simulink model "torqueBalancingStandup"  (Simulink 9.1)
settings: Solver=FixedStepDiscrete  StartTime=0.0  StopTime="Config.SIMULATION_TIME "  FixedStep=Config.Ts  RelTol=1e-3  EnableMultiTasking=on
InitFcn:
  | cd(fileparts(which(bdroot)));
  | initTorqueBalancingPHRIStandup;
StopFcn:
  | cd(fileparts(which(bdroot)));
  | stopTorqueBalancingPHRIStandup;
undefined symbols (not defined in the file or in its folder): bVectorConstraintsFeet, bVectorConstraintsLegs, Config, ConstraintsMatrixFeet, ConstraintsMatrixLegs, Gain, HUMAN_DOF_FOR_SIMULINK, Reg, ROBOT_DOF, ROBOT_DOF_FOR_SIMULINK, Sat, Sm
libraries: WBToolboxLibrary x127, simulink x4
(part 2 of 3)

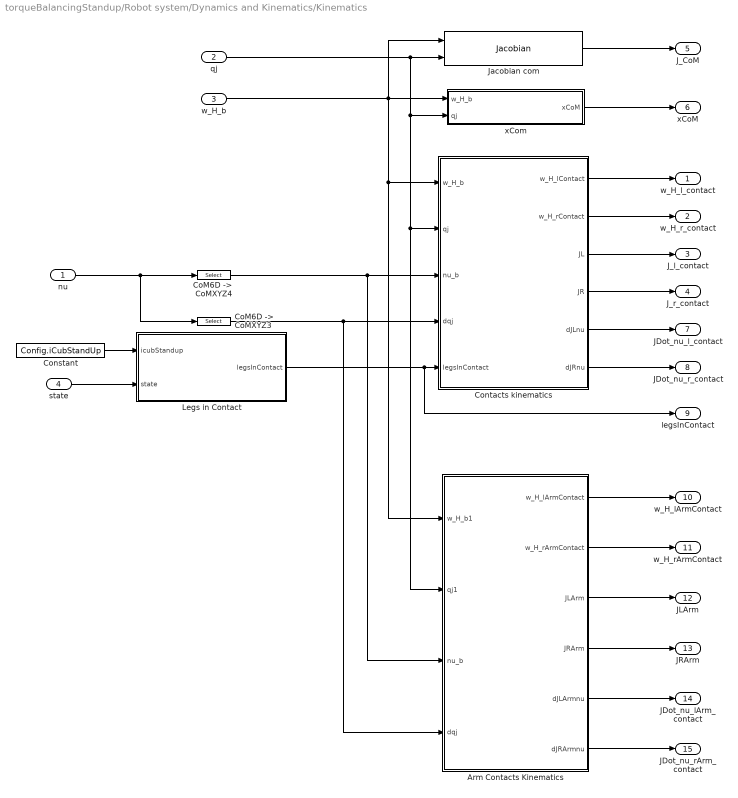
== system torqueBalancingStandup/Robot system/Dynamics and Kinematics/Kinematics ==
  nu : Inport
  qj : Inport  Port=2
  w_H_b : Inport  Port=3
  "state " : Inport  Port=4
  Arm Contacts Kinematics : Subsystem
  "CoM6D ->  CoMXYZ3" : Selector  InputPortWidth=6+ROBOT_DOF  IndexOptions=Index vector (dialog)  Indices=[7:6+ROBOT_DOF]  OutputSizes=1
  "CoM6D ->  CoMXYZ4" : Selector  InputPortWidth=6+ROBOT_DOF  IndexOptions=Index vector (dialog)  Indices=[1 2 3 4 5 6]  OutputSizes=1
  Constant : Constant  Value=Config.iCubStandUp
  Contacts kinematics : Subsystem
  Jacobian com : WBToolboxLibrary/wholeBodyModel/Jacobians/Jacobian  frameName=Frames.COM
      settings: SourceProductName=Whole Body Toolbox
  Legs in Contact : MATLAB Function  TreatAsAtomicUnit=on
  xCom : Subsystem
  w_H_l_contact : Outport
  w_H_r_contact : Outport  Port=2
  J_l_contact : Outport  Port=3
  J_r_contact : Outport  Port=4
  J_CoM : Outport  Port=5
  xCoM : Outport  Port=6
  JDot_nu_l_contact : Outport  Port=7
  JDot_nu_r_contact : Outport  Port=8
  legsInContact : Outport  Port=9
  w_H_lArmContact : Outport  Port=10
  w_H_rArmContact : Outport  Port=11
  JLArm : Outport  Port=12
  JRArm : Outport  Port=13
  JDot_nu_lArm_contact : Outport  Port=14
  JDot_nu_rArm_contact : Outport  Port=15
  wires:
  nu/1 -> "CoM6D ->  CoMXYZ3"/1, "CoM6D ->  CoMXYZ4"/1
  w_H_b/1 -> Arm Contacts Kinematics/1(w_H_b1), Contacts kinematics/1(w_H_b), xCom/1(w_H_b), Jacobian com/1
  qj/1 -> Jacobian com/2, Arm Contacts Kinematics/2(qj1), Contacts kinematics/2(qj), xCom/2(qj)
  Jacobian com/1 -> J_CoM/1
  xCom/1(xCoM) -> xCoM/1
  "state "/1 -> Legs in Contact/2(state)
  Constant/1 -> Legs in Contact/1(icubStandup)
  "CoM6D ->  CoMXYZ3"/1 -> Arm Contacts Kinematics/4(dqj), Contacts kinematics/4(dqj)
  "CoM6D ->  CoMXYZ4"/1 -> Arm Contacts Kinematics/3(nu_b), Contacts kinematics/3(nu_b)
  Legs in Contact/1(legsInContact) -> Contacts kinematics/5(legsInContact), legsInContact/1
  Contacts kinematics/1(w_H_lContact) -> w_H_l_contact/1
  Contacts kinematics/2(w_H_rContact) -> w_H_r_contact/1
  Contacts kinematics/5(dJLnu) -> JDot_nu_l_contact/1
  Contacts kinematics/6(dJRnu) -> JDot_nu_r_contact/1
  Contacts kinematics/3(JL) -> J_l_contact/1
  Contacts kinematics/4(JR) -> J_r_contact/1
  Arm Contacts Kinematics/4(JRArm) -> JRArm/1
  Arm Contacts Kinematics/5(dJLArmnu) -> JDot_nu_lArm_contact/1
  Arm Contacts Kinematics/3(JLArm) -> JLArm/1
  Arm Contacts Kinematics/1(w_H_lArmContact) -> w_H_lArmContact/1
  Arm Contacts Kinematics/6(dJRArmnu) -> JDot_nu_rArm_contact/1
  Arm Contacts Kinematics/2(w_H_rArmContact) -> w_H_rArmContact/1

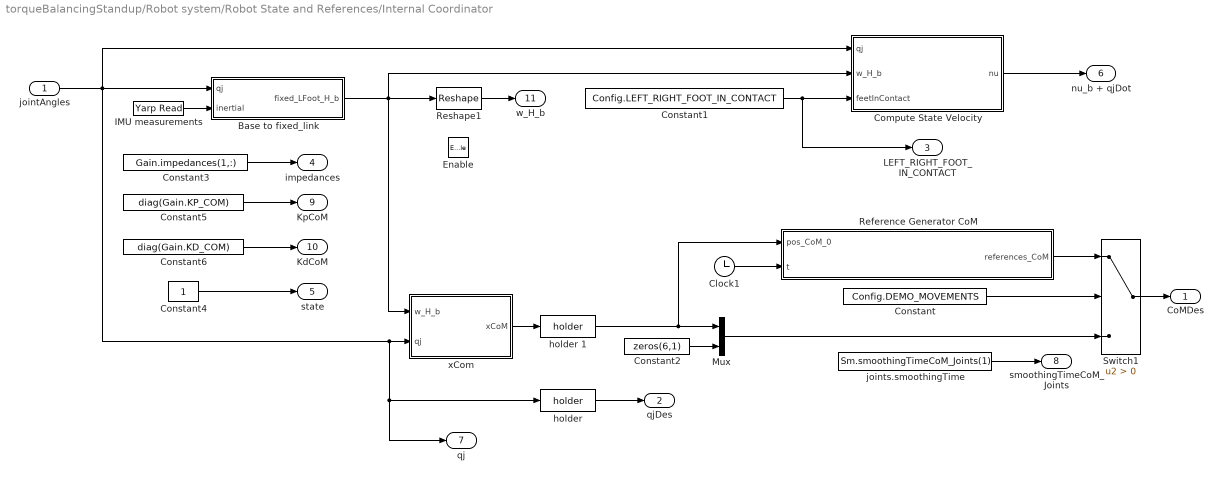
== system torqueBalancingStandup/Robot system/Robot State and References/Internal Coordinator ==
  jointAngles : Inport
  Enable : EnablePort
  Base to fixed_link : Subsystem
  Clock1 : Clock
  Compute State Velocity : Subsystem
  Constant : Constant  Value=Config.DEMO_MOVEMENTS
  Constant1 : Constant  Value=Config.LEFT_RIGHT_FOOT_IN_CONTACT
  Constant2 : Constant  Value=zeros(6,1)
  Constant3 : Constant  Value=Gain.impedances(1,:)
  Constant4 : Constant
  Constant5 : Constant  Value=diag(Gain.KP_COM)
  Constant6 : Constant  Value=diag(Gain.KD_COM)
  IMU measurements : WBToolboxLibrary/Utilities/Yarp Read  portName=Ports.IMU  signalSize=12  timeout=0.5  blocking=off  timestamp=off  autoconnect=on  errorOnConnection=on
      settings: SourceProductName=Whole Body Toolbox
  Mux : Mux  Inputs=2
  Reference Generator CoM : MATLAB Function  TreatAsAtomicUnit=on
  Reshape1 : Reshape  OutputDimensions=[4;4]
  Switch1 : Switch  Criteria=u2 > Threshold
  "holder " : WBToolboxLibrary/Utilities/holder 
      settings: SourceProductName=Whole Body Toolbox
  holder 1 : WBToolboxLibrary/Utilities/holder 
      settings: SourceProductName=Whole Body Toolbox
  joints.smoothingTime : Constant  Value=Sm.smoothingTimeCoM_Joints(1)
  xCom : Subsystem
  CoMDes : Outport
  qjDes : Outport  Port=2
  LEFT_RIGHT_FOOT_IN_CONTACT : Outport  Port=3
  impedances : Outport  Port=4
  state : Outport  Port=5
  nu_b + qjDot : Outport  Port=6
  qj : Outport  Port=7
  smoothingTimeCoM_Joints : Outport  Port=8
  KpCoM : Outport  Port=9
  KdCoM : Outport  Port=10
  w_H_b : Outport  Port=11
  wires:
  Constant/1 -> Switch1/2
  "holder "/1 -> qjDes/1
  Switch1/1 -> CoMDes/1
  Mux/1 -> Switch1/3
  Constant2/1 -> Mux/2
  Constant3/1 -> impedances/1
  Constant4/1 -> state/1
  Compute State Velocity/1(nu) -> nu_b + qjDot/1
  holder 1/1 -> Reference Generator CoM/1(pos_CoM_0), Mux/1
  Base to fixed_link/1(fixed_LFoot_H_b) -> Compute State Velocity/2(w_H_b), xCom/1(w_H_b), Reshape1/1
  xCom/1(xCoM) -> holder 1/1
  joints.smoothingTime/1 -> smoothingTimeCoM_Joints/1
  jointAngles/1 -> Compute State Velocity/1(qj), Base to fixed_link/1(qj), qj/1, "holder "/1, xCom/2(qj)
  Constant5/1 -> KpCoM/1
  Constant6/1 -> KdCoM/1
  Reshape1/1 -> w_H_b/1
  Constant1/1 -> Compute State Velocity/3("feetInContact "), LEFT_RIGHT_FOOT_IN_CONTACT/1
  IMU measurements/1 -> Base to fixed_link/2(inertial)
  Clock1/1 -> Reference Generator CoM/2(t)
  Reference Generator CoM/1(references_CoM) -> Switch1/1

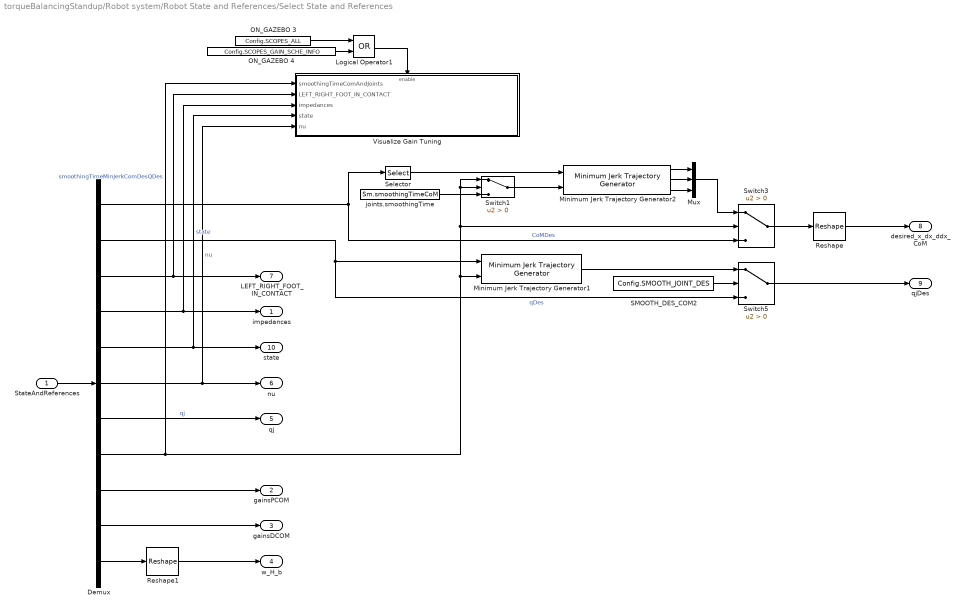
== system torqueBalancingStandup/Robot system/Robot State and References/Select State and References ==
  StateAndReferences : Inport
  Demux : Demux  Outputs=[9,ROBOT_DOF,2,ROBOT_DOF,1,ROBOT_DOF+6,ROBOT_DOF,1,3,3,16]
  Logical Operator1 : Logic  Operator=OR  AllPortsSameDT=off  OutDataTypeStr=boolean
  Minimum Jerk Trajectory Generator1 : WBToolboxLibrary/Utilities/Minimum Jerk Trajectory Generator  externalSettlingTime=on  settlingTime=1  sampleTime=Config.Ts  resetOnSettlingTime=off  firstDerivatives=off  secondDerivatives=off  explicitInitialValue=off
      settings: SourceProductName=Whole Body Toolbox
  Minimum Jerk Trajectory Generator2 : WBToolboxLibrary/Utilities/Minimum Jerk Trajectory Generator  externalSettlingTime=on  settlingTime=0.1  sampleTime=Config.Ts  resetOnSettlingTime=off  firstDerivatives=on  secondDerivatives=on  explicitInitialValue=off
      settings: SourceProductName=Whole Body Toolbox
  Mux : Mux  Inputs=3
  ON_GAZEBO 3 : Constant  Value=Config.SCOPES_ALL
  ON_GAZEBO 4 : Constant  Value=Config.SCOPES_GAIN_SCHE_INFO
  Reshape : Reshape  OutputDimensionality=Customize  OutputDimensions=[3,3]
  Reshape1 : Reshape  OutputDimensionality=Customize  OutputDimensions=[4;4]
  SMOOTH_DES_COM2 : Constant  Value=Config.SMOOTH_JOINT_DES
  Selector : Selector  InputPortWidth=9  IndexOptions=Index vector (dialog)  Indices=[1 2 3]  OutputSizes=1
  Switch1 : Switch  Criteria=u2 > Threshold
  Switch3 : Switch  Criteria=u2 > Threshold
  Switch5 : Switch  Criteria=u2 > Threshold
  "Visualize Gain Tuning  " : Subsystem
  joints.smoothingTime : Constant  Value=Sm.smoothingTimeCoM
  impedances : Outport
  gainsPCOM : Outport  Port=2
  gainsDCOM : Outport  Port=3
  w_H_b : Outport  Port=4
  qj : Outport  Port=5
  nu : Outport  Port=6
  LEFT_RIGHT_FOOT_IN_CONTACT : Outport  Port=7
  desired_x_dx_ddx_CoM : Outport  Port=8
  qjDes : Outport  Port=9
  state : Outport  Port=10
  wires:
  Reshape/1 -> desired_x_dx_ddx_CoM/1
  Minimum Jerk Trajectory Generator2/1 -> Mux/1
  Minimum Jerk Trajectory Generator2/2 -> Mux/2
  Switch3/1 -> Reshape/1
  Minimum Jerk Trajectory Generator2/3 -> Mux/3
  SMOOTH_DES_COM2/1 -> Switch5/2
  Switch5/1 -> qjDes/1
  Demux/7 -> qj/1  "qj"
  Demux/11 -> Reshape1/1
  Demux/5 -> "Visualize Gain Tuning  "/4(state), state/1  "state"
  Demux/8 -> Switch1/1, Switch1/2, Switch3/2, Minimum Jerk Trajectory Generator1/2, "Visualize Gain Tuning  "/1(smoothingTimeComAndJoints)  "smoothingTimeMinJerkComDesQDes"
  Mux/1 -> Switch3/1
  Selector/1 -> Minimum Jerk Trajectory Generator2/1
  Demux/2 -> Switch5/3, Minimum Jerk Trajectory Generator1/1  "qDes"
  Minimum Jerk Trajectory Generator1/1 -> Switch5/1
  Demux/6 -> "Visualize Gain Tuning  "/5(nu), nu/1  "nu"
  StateAndReferences/1 -> Demux/1
  Demux/4 -> "Visualize Gain Tuning  "/3(impedances), impedances/1
  Demux/3 -> "Visualize Gain Tuning  "/2(LEFT_RIGHT_FOOT_IN_CONTACT), LEFT_RIGHT_FOOT_IN_CONTACT/1
  Demux/9 -> gainsPCOM/1
  Demux/10 -> gainsDCOM/1
  Demux/1 -> Selector/1, Switch3/3  "CoMDes"
  Reshape1/1 -> w_H_b/1
  ON_GAZEBO 4/1 -> Logical Operator1/2
  ON_GAZEBO 3/1 -> Logical Operator1/1
  Logical Operator1/1 -> "Visualize Gain Tuning  "/Enable
  Switch1/1 -> Minimum Jerk Trajectory Generator2/2
  joints.smoothingTime/1 -> Switch1/3

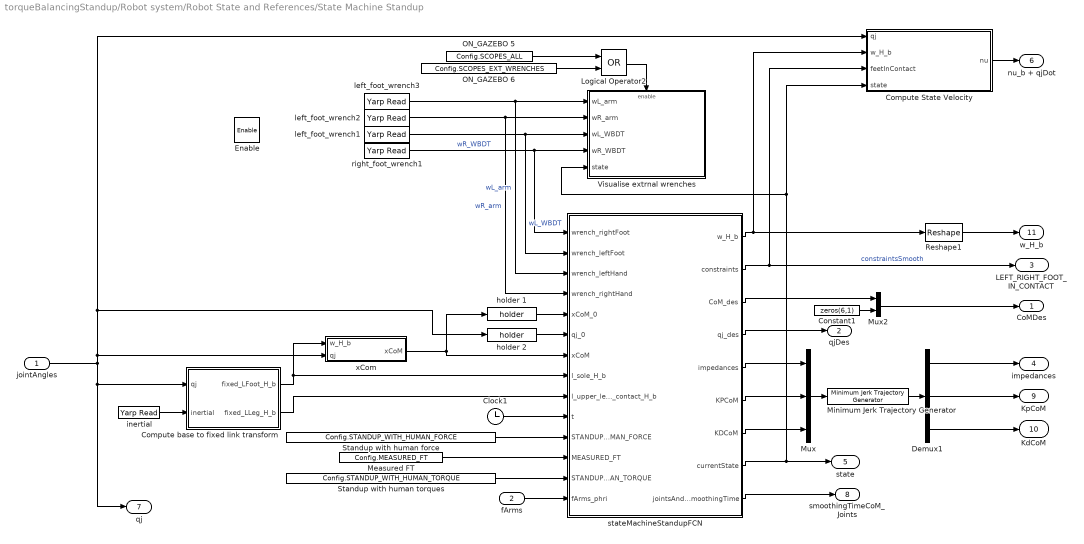
== system torqueBalancingStandup/Robot system/Robot State and References/State Machine Standup ==
  jointAngles : Inport
  fArms : Inport  Port=2
  Enable : EnablePort
  Clock1 : Clock
  Compute State Velocity : Subsystem
  Compute base to fixed link transform : Subsystem
  Constant1 : Constant  Value=zeros(6,1)
  Demux1 : Demux  Outputs=[ROBOT_DOF,3,3]
  Logical Operator2 : Logic  Operator=OR  AllPortsSameDT=off  OutDataTypeStr=boolean
  Measured FT : Constant  Value=Config.MEASURED_FT
  Minimum Jerk Trajectory Generator : WBToolboxLibrary/Utilities/Minimum Jerk Trajectory Generator  externalSettlingTime=off  settlingTime=Gain.SmoothingTimeGainScheduling  sampleTime=Config.Ts  resetOnSettlingTime=off  firstDerivatives=off  secondDerivatives=off  explicitInitialValue=off
      settings: SourceProductName=Whole Body Toolbox
  Mux : Mux  Inputs=3
  Mux2 : Mux  Inputs=2
  ON_GAZEBO 5 : Constant  Value=Config.SCOPES_ALL
  ON_GAZEBO 6 : Constant  Value=Config.SCOPES_EXT_WRENCHES
  Reshape1 : Reshape  OutputDimensions=[4;4]
  Standup with human force : Constant  Value=Config.STANDUP_WITH_HUMAN_FORCE
  Standup with human torques : Constant  Value=Config.STANDUP_WITH_HUMAN_TORQUE
  Visualise extrnal wrenches : Subsystem
  holder 1 : WBToolboxLibrary/Utilities/holder 
      settings: SourceProductName=Whole Body Toolbox
  holder 2 : WBToolboxLibrary/Utilities/holder 
      settings: SourceProductName=Whole Body Toolbox
  inertial : WBToolboxLibrary/Utilities/Yarp Read  portName=Ports.IMU  signalSize=12  timeout=0.5  blocking=off  timestamp=off  autoconnect=on  errorOnConnection=off
      settings: SourceProductName=Whole Body Toolbox
  left_foot_wrench1 : WBToolboxLibrary/Utilities/Yarp Read  portName=Ports.WBD_LEFTLEG_EE  signalSize=6  timeout=0.5  blocking=off  timestamp=off  autoconnect=on  errorOnConnection=on
      settings: SourceProductName=Whole Body Toolbox
  left_foot_wrench2 : WBToolboxLibrary/Utilities/Yarp Read  portName=Ports.RIGHT_ARM  signalSize=6  timeout=0.5  blocking=off  timestamp=off  autoconnect=on  errorOnConnection=on
      settings: SourceProductName=Whole Body Toolbox
  left_foot_wrench3 : WBToolboxLibrary/Utilities/Yarp Read  portName=Ports.LEFT_ARM  signalSize=6  timeout=0.5  blocking=off  timestamp=off  autoconnect=on  errorOnConnection=on
      settings: SourceProductName=Whole Body Toolbox
  right_foot_wrench1 : WBToolboxLibrary/Utilities/Yarp Read  portName=Ports.WBD_RIGHTLEG_EE  signalSize=6  timeout=0.5  blocking=off  timestamp=off  autoconnect=on  errorOnConnection=on
      settings: SourceProductName=Whole Body Toolbox
  stateMachineStandupFCN : MATLAB Function  TreatAsAtomicUnit=on
  xCom : Subsystem
  CoMDes : Outport
  qjDes : Outport  Port=2
  LEFT_RIGHT_FOOT_IN_CONTACT : Outport  Port=3
  impedances : Outport  Port=4
  state : Outport  Port=5
  nu_b + qjDot : Outport  Port=6
  qj : Outport  Port=7
  smoothingTimeCoM_Joints : Outport  Port=8
  KpCoM : Outport  Port=9
  KdCoM : Outport  Port=10
  w_H_b : Outport  Port=11
  wires:
  xCom/1(xCoM) -> holder 1/1, stateMachineStandupFCN/7(xCoM)
  stateMachineStandupFCN/4(qj_des) -> qjDes/1
  stateMachineStandupFCN/3(CoM_des) -> Mux2/1
  Mux2/1 -> CoMDes/1
  Constant1/1 -> Mux2/2
  stateMachineStandupFCN/8(currentState) -> Visualise extrnal wrenches/5(state), Compute State Velocity/4("state "), state/1
  stateMachineStandupFCN/2(constraints) -> LEFT_RIGHT_FOOT_IN_CONTACT/1, Compute State Velocity/3("feetInContact ")  "constraintsSmooth"
  stateMachineStandupFCN/1(w_H_b) -> Reshape1/1, Compute State Velocity/2(w_H_b)
  Compute State Velocity/1(nu) -> nu_b + qjDot/1
  stateMachineStandupFCN/9(jointsAndCoMSmoothingTime) -> smoothingTimeCoM_Joints/1
  stateMachineStandupFCN/6(KPCoM) -> Mux/2
  Demux1/3 -> KdCoM/1
  stateMachineStandupFCN/7(KDCoM) -> Mux/3
  stateMachineStandupFCN/5(impedances) -> Mux/1
  Mux/1 -> Minimum Jerk Trajectory Generator/1
  Minimum Jerk Trajectory Generator/1 -> Demux1/1
  Demux1/1 -> impedances/1
  Demux1/2 -> KpCoM/1
  jointAngles/1 -> Compute State Velocity/1(qj), holder 2/1, xCom/2(qj), qj/1, Compute base to fixed link transform/1(qj)
  Compute base to fixed link transform/1(fixed_LFoot_H_b) -> xCom/1(w_H_b), stateMachineStandupFCN/8(l_sole_H_b)
  Compute base to fixed link transform/2(fixed_LLeg_H_b) -> stateMachineStandupFCN/9(l_upper_leg_contact_H_b)
  inertial/1 -> Compute base to fixed link transform/2(inertial)
  Reshape1/1 -> w_H_b/1
  right_foot_wrench1/1 -> stateMachineStandupFCN/1(wrench_rightFoot), Visualise extrnal wrenches/4(wR_WBDT)  "wR_WBDT"
  left_foot_wrench1/1 -> stateMachineStandupFCN/2(wrench_leftFoot), Visualise extrnal wrenches/3(wL_WBDT)  "wL_WBDT"
  Logical Operator2/1 -> Visualise extrnal wrenches/Enable
  ON_GAZEBO 5/1 -> Logical Operator2/1
  ON_GAZEBO 6/1 -> Logical Operator2/2
  left_foot_wrench2/1 -> stateMachineStandupFCN/4(wrench_rightHand), Visualise extrnal wrenches/2(wR_arm)  "wR_arm"
  left_foot_wrench3/1 -> stateMachineStandupFCN/3(wrench_leftHand), Visualise extrnal wrenches/1(wL_arm)  "wL_arm"
  holder 1/1 -> stateMachineStandupFCN/5(xCoM_0)
  holder 2/1 -> stateMachineStandupFCN/6(qj_0)
  Clock1/1 -> stateMachineStandupFCN/10(t)
  Measured FT/1 -> stateMachineStandupFCN/12(MEASURED_FT)
  fArms/1 -> stateMachineStandupFCN/14(fArms_phri)
  Standup with human force/1 -> stateMachineStandupFCN/11(STANDUP_WITH_HUMAN_FORCE)
  Standup with human torques/1 -> stateMachineStandupFCN/13(STANDUP_WITH_HUMAN_TORQUE)

== system torqueBalancingStandup/Robot system/controller_QP/Compute angular momentum integral ==
  qjDes : Inport
  qj : Inport  Port=2
  constraints : Inport  Port=3
  state : Inport  Port=4
  Centroidal Momentum : WBToolboxLibrary/wholeBodyModel/Dynamics/Centroidal Momentum
      settings: SourceProductName=Whole Body Toolbox
  Compute base to fixed link transform : Subsystem
  Constant : Constant  Value=Config.iCubStandUp
  Fixed Links Jacobians : Subsystem
  Legs in Contact : MATLAB Function  TreatAsAtomicUnit=on
  References for H : MATLAB Function  TreatAsAtomicUnit=on
  Selector : Selector  InputPortWidth=6  IndexOptions=Index vector (dialog)  Indices=[4 5 6]  OutputSizes=1
  Sum : Sum  Inputs=|-+
  Switch : Switch  Criteria=u2 > Threshold  Threshold=0.1
  inertial : WBToolboxLibrary/Utilities/Yarp Read  portName=Ports.IMU  signalSize=12  timeout=0.5  blocking=off  timestamp=off  autoconnect=on  errorOnConnection=on
      settings: SourceProductName=Whole Body Toolbox
  intHw : Outport
  wires:
  qjDes/1 -> Sum/1, Compute base to fixed link transform/1(qj), Fixed Links Jacobians/2(qj), Centroidal Momentum/2
  qj/1 -> Sum/2
  Sum/1 -> Centroidal Momentum/4, References for H/1(qjErr)
  References for H/1(nu_b_equivalent) -> Centroidal Momentum/3
  Fixed Links Jacobians/1(J_LeftFixed) -> References for H/2(JL)
  Centroidal Momentum/1 -> Selector/1
  Selector/1 -> intHw/1
  Fixed Links Jacobians/2(J_RIghtFixed) -> References for H/3(JR)
  constraints/1 -> References for H/4(activeFeetConstraints)
  Switch/1 -> Centroidal Momentum/1, Fixed Links Jacobians/3(w_H_b)
  inertial/1 -> Compute base to fixed link transform/2(inertial)
  state/1 -> Legs in Contact/2(state)
  Constant/1 -> Legs in Contact/1(icubStandup)
  Legs in Contact/1(legsInContact) -> Fixed Links Jacobians/1("legsInContact "), Switch/2
  Compute base to fixed link transform/1(fixed_LLeg_H_b) -> Switch/1
  Compute base to fixed link transform/2(fixed_LFoot_H_b) -> Switch/3

== system torqueBalancingStandup/Robot system/controller_QP/Compute joint torques ==
  LEFT_RIGHT_FOOT_IN_CONTACT : Inport
  tauModel : Inport  Port=2
  Sigma : Inport  Port=3
  NA : Inport  Port=4
  fHDes : Inport  Port=5
  HessianMatrixQP1Foot : Inport  Port=6
  gradientQP1Foot : Inport  Port=7
  ConstraintsMatrixQP1Foot : Inport  Port=8
  bVectorConstraintsQP1Foot : Inport  Port=9
  HessianMatrixQP2Feet : Inport  Port=10
  gradientQP2Feet : Inport  Port=11
  ConstraintsMatrixQP2Feet : Inport  Port=12
  bVectorConstraintsQp2Feet : Inport  Port=13
  state : Inport  Port=14
  Add : Sum
  Add1 : Sum
  Product1 : Product  Multiplication=Matrix(*)
  Product2 : Product  Multiplication=Matrix(*)
  QPSolver : Subsystem
  Sum : Sum  Inputs=|++
  "tau " : Outport
  fDes QP : Outport  Port=2
  wires:
  NA/1 -> Product2/1
  QPSolver/1(f0OneFoot) -> Sum/2
  Product1/1 -> Add/2
  tauModel/1 -> Add/1
  Add/1 -> "tau "/1
  Add1/1 -> fDes QP/1, Product1/2
  Sum/1 -> Add1/1
  Product2/1 -> Add1/2
  Sigma/1 -> Product1/1
  QPSolver/2(f0TwoFeet) -> Product2/2
  gradientQP1Foot/1 -> QPSolver/3(gradientQP1Foot)
  ConstraintsMatrixQP2Feet/1 -> QPSolver/8(ConstraintsMatrixQP2Feet)
  LEFT_RIGHT_FOOT_IN_CONTACT/1 -> QPSolver/1(LEFT_RIGHT_FOOT_IN_CONTACT)
  bVectorConstraintsQP1Foot/1 -> QPSolver/5(bVectorConstraintsQP1Foot)
  HessianMatrixQP1Foot/1 -> QPSolver/2(HessianMatrixQP1Foot)
  ConstraintsMatrixQP1Foot/1 -> QPSolver/4(ConstraintsMatrixQP1Foot)
  gradientQP2Feet/1 -> QPSolver/7(gradientQP2Feet)
  HessianMatrixQP2Feet/1 -> QPSolver/6(HessianMatrixQP2Feet)
  bVectorConstraintsQp2Feet/1 -> QPSolver/9(bVectorConstraintsQp2Feet)
  state/1 -> QPSolver/10(state)
  fHDes/1 -> Sum/1

== system torqueBalancingStandup/Robot system/controller_QP/Compute joint torques (motor reflected inertia) ==
  u : Inport
  " " : Constant  Value=Config.USE_MOTOR_REFLECTED_INERTIA
  "(transpose(T*Gamma))^{-1}*I_m*(T*Gamma)^{-1}" : MATLAB Function  TreatAsAtomicUnit=on
  Add : Sum  Inputs=-+
  Gain : Gain  Gain=Config.K_ff
  Get Measurement : WBToolboxLibrary/wholeBodyStates/Get Measurement  measuredType=Joints Acceleration
      settings: SourceProductName=Whole Body Toolbox
  Product : Product  Multiplication=Matrix(*)
  Switch : Switch  Criteria=u2 > Threshold
  tau_joints : Outport
  wires:
  Get Measurement/1 -> Product/2
  Product/1 -> Gain/1
  Gain/1 -> Add/1
  Add/1 -> Switch/1
  " "/1 -> Switch/2
  Switch/1 -> tau_joints/1
  u/1 -> Add/2, Switch/3
  "(transpose(T*Gamma))^{-1}*I_m*(T*Gamma)^{-1}"/1(reflectedInertia) -> Product/1

== system torqueBalancingStandup/Robot system/controller_QP/Constraints ==
  legsInContact : Inport
  Constant : Constant  Value=ConstraintsMatrixFeet
  Constant1 : Constant  Value=bVectorConstraintsLegs
  Constant2 : Constant  Value=ConstraintsMatrixLegs
  Constant3 : Constant  Value=bVectorConstraintsFeet
  Switch1 : Switch  Criteria=u2 > Threshold  Threshold=0.1
  Switch2 : Switch  Criteria=u2 > Threshold  Threshold=0.1
  ConstraintsMatrix : Outport
  bVectorConstraints : Outport  Port=2
  wires:
  Constant2/1 -> Switch1/1
  Constant/1 -> Switch1/3
  Constant1/1 -> Switch2/1
  Constant3/1 -> Switch2/3
  legsInContact/1 -> Switch2/2, Switch1/2
  Switch1/1 -> ConstraintsMatrix/1
  Switch2/1 -> bVectorConstraints/1

== system torqueBalancingStandup/Robot system/synchronizer/GAZEBO_SYNCHRONIZER ==
  Enable : EnablePort
  Simulator Synchronizer : WBToolboxLibrary/Utilities/Simulator Synchronizer  period=Config.Ts  serverPortName='/clock/rpc'  clientPortName='/WBT_synchronizer/rpc:o'
      settings: SourceProductName=Whole Body Toolbox

== system torqueBalancingStandup/Robot system/synchronizer/REAL_TIME_SYNC ==
  Enable : EnablePort
  Real Time Synchronizer : WBToolboxLibrary/Utilities/Real Time Synchronizer  period=Config.Ts
      settings: SourceProductName=Whole Body Toolbox

== system torqueBalancingStandup/Human system/Dump and visualize/Human data/human joint data ==
  human_jointData : Inport
  Scope : Scope  NumInputPorts=6
  head : Selector  InputPortWidth=66  IndexOptions=Index vector (dialog)  Indices=[16 17 18]  OutputSizes=1
  jointData : Scope  NumInputPorts=16
  left_ankle : Selector  InputPortWidth=66  IndexOptions=Index vector (dialog)  Indices=[61 62 63]  OutputSizes=1
  left_ball_foot : Selector  InputPortWidth=66  IndexOptions=Index vector (dialog)  Indices=[64 65 66]  OutputSizes=1
  left_elbow : Selector  InputPortWidth=66  IndexOptions=Index vector (dialog)  Indices=[37 38 39]  OutputSizes=1
  left_hip : Selector  InputPortWidth=66  IndexOptions=Index vector (dialog)  Indices=[55 56 57]  OutputSizes=1
  left_knee : Selector  InputPortWidth=66  IndexOptions=Index vector (dialog)  Indices=[58 59 60]  OutputSizes=1
  left_shoulder : Selector  InputPortWidth=66  IndexOptions=Index vector (dialog)  Indices=[34 35 36]  OutputSizes=1
  left_shoulder_internal : Selector  InputPortWidth=66  IndexOptions=Index vector (dialog)  Indices=[31 32 33]  OutputSizes=1
  left_wrist : Selector  InputPortWidth=66  IndexOptions=Index vector (dialog)  Indices=[40 41 42]  OutputSizes=1
  neck : Selector  InputPortWidth=66  IndexOptions=Index vector (dialog)  Indices=[13 14 15]  OutputSizes=1
  right_ankle : Selector  InputPortWidth=66  IndexOptions=Index vector (dialog)  Indices=[49 50 51]  OutputSizes=1
  right_ball_foot : Selector  InputPortWidth=66  IndexOptions=Index vector (dialog)  Indices=[52 53 54]  OutputSizes=1
  right_elbow : Selector  InputPortWidth=66  IndexOptions=Index vector (dialog)  Indices=[25 26 27]  OutputSizes=1
  right_hip : Selector  InputPortWidth=66  IndexOptions=Index vector (dialog)  Indices=[43 44 45]  OutputSizes=1
  right_knee : Selector  InputPortWidth=66  IndexOptions=Index vector (dialog)  Indices=[46 47 48]  OutputSizes=1
  right_shoulder : Selector  InputPortWidth=66  IndexOptions=Index vector (dialog)  Indices=[22 23 24]  OutputSizes=1
  right_shoulder_internal : Selector  InputPortWidth=66  IndexOptions=Index vector (dialog)  Indices=[19 20 21]  OutputSizes=1
  right_wrist : Selector  InputPortWidth=66  IndexOptions=Index vector (dialog)  Indices=[28 29 30]  OutputSizes=1
  torso_1 : Selector  InputPortWidth=66  IndexOptions=Index vector (dialog)  Indices=[10 11 12]  OutputSizes=1
  torso_2 : Selector  InputPortWidth=66  IndexOptions=Index vector (dialog)  Indices=[7 8 9]  OutputSizes=1
  torso_3 : Selector  InputPortWidth=66  IndexOptions=Index vector (dialog)  Indices=[4 5 6]  OutputSizes=1
  torso_4 : Selector  InputPortWidth=66  IndexOptions=Index vector (dialog)  Indices=[1 2 3]  OutputSizes=1
  wires:
  torso_1/1 -> jointData/1
  torso_4/1 -> jointData/4
  torso_3/1 -> jointData/3
  torso_2/1 -> jointData/2
  right_shoulder_internal/1 -> jointData/6
  left_shoulder_internal/1 -> jointData/5
  left_hip/1 -> jointData/7
  right_hip/1 -> jointData/8
  left_shoulder/1 -> jointData/9
  right_shoulder/1 -> jointData/10
  left_knee/1 -> jointData/11
  right_knee/1 -> jointData/12
  left_elbow/1 -> jointData/13
  right_elbow/1 -> jointData/14
  left_ankle/1 -> jointData/15
  right_ankle/1 -> jointData/16
  human_jointData/1 -> head/1, left_ball_foot/1, left_wrist/1, neck/1, right_ball_foot/1, right_wrist/1, left_shoulder/1, right_hip/1, left_hip/1, right_shoulder_internal/1, torso_1/1, torso_2/1, torso_3/1, torso_4/1, left_shoulder_internal/1, right_shoulder/1, left_knee/1, right_knee/1, left_elbow/1, right_elbow/1, right_ankle/1, left_ankle/1
  head/1 -> Scope/1
  left_ball_foot/1 -> Scope/2
  left_wrist/1 -> Scope/3
  neck/1 -> Scope/4
  right_ball_foot/1 -> Scope/5
  right_wrist/1 -> Scope/6

== system torqueBalancingStandup/Human system/Dump and visualize/Human data/human joint torques data ==
  human_jointTorquesData : Inport
  Scope : Scope  NumInputPorts=6
  head : Selector  InputPortWidth=66  IndexOptions=Index vector (dialog)  Indices=[16 17 18]  OutputSizes=1
  jointTorquesData : Scope  NumInputPorts=16
  left_ankle : Selector  InputPortWidth=66  IndexOptions=Index vector (dialog)  Indices=[61 62 63]  OutputSizes=1
  left_ball_foot : Selector  InputPortWidth=66  IndexOptions=Index vector (dialog)  Indices=[64 65 66]  OutputSizes=1
  left_elbow : Selector  InputPortWidth=66  IndexOptions=Index vector (dialog)  Indices=[37 38 39]  OutputSizes=1
  left_hip : Selector  InputPortWidth=66  IndexOptions=Index vector (dialog)  Indices=[55 56 57]  OutputSizes=1
  left_knee : Selector  InputPortWidth=66  IndexOptions=Index vector (dialog)  Indices=[58 59 60]  OutputSizes=1
  left_shoulder : Selector  InputPortWidth=66  IndexOptions=Index vector (dialog)  Indices=[34 35 36]  OutputSizes=1
  left_shoulder_internal : Selector  InputPortWidth=66  IndexOptions=Index vector (dialog)  Indices=[31 32 33]  OutputSizes=1
  left_wrist : Selector  InputPortWidth=66  IndexOptions=Index vector (dialog)  Indices=[40 41 42]  OutputSizes=1
  neck : Selector  InputPortWidth=66  IndexOptions=Index vector (dialog)  Indices=[13 14 15]  OutputSizes=1
  right_ankle : Selector  InputPortWidth=66  IndexOptions=Index vector (dialog)  Indices=[49 50 51]  OutputSizes=1
  right_ball_foot : Selector  InputPortWidth=66  IndexOptions=Index vector (dialog)  Indices=[52 53 54]  OutputSizes=1
  right_elbow : Selector  InputPortWidth=66  IndexOptions=Index vector (dialog)  Indices=[25 26 27]  OutputSizes=1
  right_hip : Selector  InputPortWidth=66  IndexOptions=Index vector (dialog)  Indices=[43 44 45]  OutputSizes=1
  right_knee : Selector  InputPortWidth=66  IndexOptions=Index vector (dialog)  Indices=[46 47 48]  OutputSizes=1
  right_shoulder : Selector  InputPortWidth=66  IndexOptions=Index vector (dialog)  Indices=[22 23 24]  OutputSizes=1
  right_shoulder_internal : Selector  InputPortWidth=66  IndexOptions=Index vector (dialog)  Indices=[19 20 21]  OutputSizes=1
  right_wrist : Selector  InputPortWidth=66  IndexOptions=Index vector (dialog)  Indices=[28 29 30]  OutputSizes=1
  torso_1 : Selector  InputPortWidth=66  IndexOptions=Index vector (dialog)  Indices=[10 11 12]  OutputSizes=1
  torso_2 : Selector  InputPortWidth=66  IndexOptions=Index vector (dialog)  Indices=[7 8 9]  OutputSizes=1
  torso_3 : Selector  InputPortWidth=66  IndexOptions=Index vector (dialog)  Indices=[4 5 6]  OutputSizes=1
  torso_4 : Selector  InputPortWidth=66  IndexOptions=Index vector (dialog)  Indices=[1 2 3]  OutputSizes=1
  wires:
  torso_1/1 -> jointTorquesData/1
  torso_4/1 -> jointTorquesData/4
  torso_3/1 -> jointTorquesData/3
  torso_2/1 -> jointTorquesData/2
  right_shoulder_internal/1 -> jointTorquesData/6
  left_shoulder_internal/1 -> jointTorquesData/5
  left_hip/1 -> jointTorquesData/7
  right_hip/1 -> jointTorquesData/8
  left_shoulder/1 -> jointTorquesData/9
  right_shoulder/1 -> jointTorquesData/10
  left_knee/1 -> jointTorquesData/11
  right_knee/1 -> jointTorquesData/12
  left_elbow/1 -> jointTorquesData/13
  right_elbow/1 -> jointTorquesData/14
  left_ankle/1 -> jointTorquesData/15
  right_ankle/1 -> jointTorquesData/16
  human_jointTorquesData/1 -> head/1, left_ball_foot/1, left_wrist/1, neck/1, right_ball_foot/1, right_wrist/1, left_shoulder/1, right_hip/1, left_hip/1, right_shoulder_internal/1, torso_1/1, torso_2/1, torso_3/1, torso_4/1, left_shoulder_internal/1, right_shoulder/1, left_knee/1, right_knee/1, left_elbow/1, right_elbow/1, right_ankle/1, left_ankle/1
  head/1 -> Scope/1
  left_ball_foot/1 -> Scope/2
  left_wrist/1 -> Scope/3
  neck/1 -> Scope/4
  right_ball_foot/1 -> Scope/5
  right_wrist/1 -> Scope/6

== system torqueBalancingStandup/Human system/Dump and visualize/Human data/human joint velocities data ==
  human_jointVelocitiesData : Inport
  Scope : Scope  NumInputPorts=6
  head : Selector  InputPortWidth=66  IndexOptions=Index vector (dialog)  Indices=[16 17 18]  OutputSizes=1
  jointVelocitiesData : Scope  NumInputPorts=16
  left_ankle : Selector  InputPortWidth=66  IndexOptions=Index vector (dialog)  Indices=[61 62 63]  OutputSizes=1
  left_ball_foot : Selector  InputPortWidth=66  IndexOptions=Index vector (dialog)  Indices=[64 65 66]  OutputSizes=1
  left_elbow : Selector  InputPortWidth=66  IndexOptions=Index vector (dialog)  Indices=[37 38 39]  OutputSizes=1
  left_hip : Selector  InputPortWidth=66  IndexOptions=Index vector (dialog)  Indices=[55 56 57]  OutputSizes=1
  left_knee : Selector  InputPortWidth=66  IndexOptions=Index vector (dialog)  Indices=[58 59 60]  OutputSizes=1
  left_shoulder : Selector  InputPortWidth=66  IndexOptions=Index vector (dialog)  Indices=[34 35 36]  OutputSizes=1
  left_shoulder_internal : Selector  InputPortWidth=66  IndexOptions=Index vector (dialog)  Indices=[31 32 33]  OutputSizes=1
  left_wrist : Selector  InputPortWidth=66  IndexOptions=Index vector (dialog)  Indices=[40 41 42]  OutputSizes=1
  neck : Selector  InputPortWidth=66  IndexOptions=Index vector (dialog)  Indices=[13 14 15]  OutputSizes=1
  right_ankle : Selector  InputPortWidth=66  IndexOptions=Index vector (dialog)  Indices=[49 50 51]  OutputSizes=1
  right_ball_foot : Selector  InputPortWidth=66  IndexOptions=Index vector (dialog)  Indices=[52 53 54]  OutputSizes=1
  right_elbow : Selector  InputPortWidth=66  IndexOptions=Index vector (dialog)  Indices=[25 26 27]  OutputSizes=1
  right_hip : Selector  InputPortWidth=66  IndexOptions=Index vector (dialog)  Indices=[43 44 45]  OutputSizes=1
  right_knee : Selector  InputPortWidth=66  IndexOptions=Index vector (dialog)  Indices=[46 47 48]  OutputSizes=1
  right_shoulder : Selector  InputPortWidth=66  IndexOptions=Index vector (dialog)  Indices=[22 23 24]  OutputSizes=1
  right_shoulder_internal : Selector  InputPortWidth=66  IndexOptions=Index vector (dialog)  Indices=[19 20 21]  OutputSizes=1
  right_wrist : Selector  InputPortWidth=66  IndexOptions=Index vector (dialog)  Indices=[28 29 30]  OutputSizes=1
  torso_1 : Selector  InputPortWidth=66  IndexOptions=Index vector (dialog)  Indices=[10 11 12]  OutputSizes=1
  torso_2 : Selector  InputPortWidth=66  IndexOptions=Index vector (dialog)  Indices=[7 8 9]  OutputSizes=1
  torso_3 : Selector  InputPortWidth=66  IndexOptions=Index vector (dialog)  Indices=[4 5 6]  OutputSizes=1
  torso_4 : Selector  InputPortWidth=66  IndexOptions=Index vector (dialog)  Indices=[1 2 3]  OutputSizes=1
  wires:
  torso_1/1 -> jointVelocitiesData/1
  torso_4/1 -> jointVelocitiesData/4
  torso_3/1 -> jointVelocitiesData/3
  torso_2/1 -> jointVelocitiesData/2
  right_shoulder_internal/1 -> jointVelocitiesData/6
  left_shoulder_internal/1 -> jointVelocitiesData/5
  left_hip/1 -> jointVelocitiesData/7
  right_hip/1 -> jointVelocitiesData/8
  left_shoulder/1 -> jointVelocitiesData/9
  right_shoulder/1 -> jointVelocitiesData/10
  left_knee/1 -> jointVelocitiesData/11
  right_knee/1 -> jointVelocitiesData/12
  left_elbow/1 -> jointVelocitiesData/13
  right_elbow/1 -> jointVelocitiesData/14
  left_ankle/1 -> jointVelocitiesData/15
  right_ankle/1 -> jointVelocitiesData/16
  human_jointVelocitiesData/1 -> head/1, left_ball_foot/1, left_wrist/1, neck/1, right_ball_foot/1, right_wrist/1, left_shoulder/1, right_hip/1, left_hip/1, right_shoulder_internal/1, torso_1/1, torso_2/1, torso_3/1, torso_4/1, left_shoulder_internal/1, right_shoulder/1, left_knee/1, right_knee/1, left_elbow/1, right_elbow/1, right_ankle/1, left_ankle/1
  head/1 -> Scope/1
  left_ball_foot/1 -> Scope/2
  left_wrist/1 -> Scope/3
  neck/1 -> Scope/4
  right_ball_foot/1 -> Scope/5
  right_wrist/1 -> Scope/6

== system torqueBalancingStandup/Robot system/Dynamics and Kinematics/Dynamics/Add motors reflected inertias ==
  M : Inport
  Add motor reflected inertias : MATLAB Function  TreatAsAtomicUnit=on
  M_with_motor_inertia : Outport
  wires:
  M/1 -> Add motor reflected inertias/1(M)
  Add motor reflected inertias/1(M_with_inertia) -> M_with_motor_inertia/1

== system torqueBalancingStandup/Robot system/Dynamics and Kinematics/Kinematics/Arm Contacts Kinematics ==
  w_H_b1 : Inport
  qj1 : Inport  Port=2
  nu_b : Inport  Port=3
  dqj : Inport  Port=4
  " " : WBToolboxLibrary/wholeBodyModel/Jacobians/DotJ Nu  frameName=Frames.RIGHT_HAND
      settings: SourceProductName=Whole Body Toolbox
  "DotJ Nu l_sole " : WBToolboxLibrary/wholeBodyModel/Jacobians/DotJ Nu  frameName=Frames.LEFT_HAND
      settings: SourceProductName=Whole Body Toolbox
  Jacobian l_sole1 : WBToolboxLibrary/wholeBodyModel/Jacobians/Jacobian  frameName=Frames.LEFT_HAND
      settings: SourceProductName=Whole Body Toolbox
  Jacobian r_sole1 : WBToolboxLibrary/wholeBodyModel/Jacobians/Jacobian  frameName=Frames.RIGHT_HAND
      settings: SourceProductName=Whole Body Toolbox
  l_sole1 : WBToolboxLibrary/wholeBodyModel/Kinematics/Forward Kinematics  frameName=Frames.LEFT_HAND
      settings: SourceProductName=Whole Body Toolbox
  r_sole1 : WBToolboxLibrary/wholeBodyModel/Kinematics/Forward Kinematics  frameName=Frames.RIGHT_HAND
      settings: SourceProductName=Whole Body Toolbox
  w_H_lArmContact : Outport
  w_H_rArmContact : Outport  Port=2
  JLArm : Outport  Port=3
  JRArm : Outport  Port=4
  dJLArmnu : Outport  Port=5
  dJRArmnu : Outport  Port=6
  wires:
  w_H_b1/1 -> Jacobian l_sole1/1, " "/1, "DotJ Nu l_sole "/1, Jacobian r_sole1/1, r_sole1/1, l_sole1/1
  r_sole1/1 -> w_H_rArmContact/1
  dqj/1 -> "DotJ Nu l_sole "/4, " "/4
  nu_b/1 -> "DotJ Nu l_sole "/3, " "/3
  " "/1 -> dJRArmnu/1
  l_sole1/1 -> w_H_lArmContact/1
  Jacobian r_sole1/1 -> JRArm/1
  qj1/1 -> Jacobian l_sole1/2, " "/2, "DotJ Nu l_sole "/2, Jacobian r_sole1/2, r_sole1/2, l_sole1/2
  Jacobian l_sole1/1 -> JLArm/1
  "DotJ Nu l_sole "/1 -> dJLArmnu/1

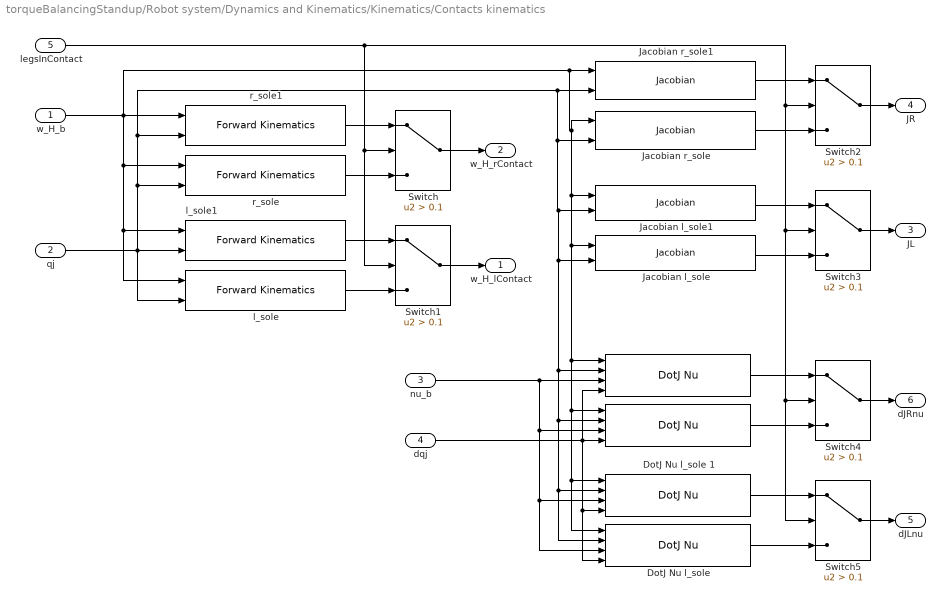
== system torqueBalancingStandup/Robot system/Dynamics and Kinematics/Kinematics/Contacts kinematics ==
  w_H_b : Inport
  qj : Inport  Port=2
  nu_b : Inport  Port=3
  dqj : Inport  Port=4
  legsInContact : Inport  Port=5
  " " : WBToolboxLibrary/wholeBodyModel/Jacobians/DotJ Nu  frameName=Frames.RIGHT_LEG
      settings: SourceProductName=Whole Body Toolbox
  "    " : WBToolboxLibrary/wholeBodyModel/Jacobians/DotJ Nu  frameName=Frames.RIGHT_FOOT
      settings: SourceProductName=Whole Body Toolbox
  "DotJ Nu l_sole " : WBToolboxLibrary/wholeBodyModel/Jacobians/DotJ Nu  frameName=Frames.LEFT_FOOT
      settings: SourceProductName=Whole Body Toolbox
  DotJ Nu l_sole 1 : WBToolboxLibrary/wholeBodyModel/Jacobians/DotJ Nu  frameName=Frames.LEFT_LEG
      settings: SourceProductName=Whole Body Toolbox
  Jacobian l_sole : WBToolboxLibrary/wholeBodyModel/Jacobians/Jacobian  frameName=Frames.LEFT_FOOT
      settings: SourceProductName=Whole Body Toolbox
  Jacobian l_sole1 : WBToolboxLibrary/wholeBodyModel/Jacobians/Jacobian  frameName=Frames.LEFT_LEG
      settings: SourceProductName=Whole Body Toolbox
  Jacobian r_sole : WBToolboxLibrary/wholeBodyModel/Jacobians/Jacobian  frameName=Frames.RIGHT_FOOT
      settings: SourceProductName=Whole Body Toolbox
  Jacobian r_sole1 : WBToolboxLibrary/wholeBodyModel/Jacobians/Jacobian  frameName=Frames.RIGHT_LEG
      settings: SourceProductName=Whole Body Toolbox
  Switch{,1..5} (6 alike) : Switch  Criteria=u2 > Threshold  Threshold=0.1
  l_sole : WBToolboxLibrary/wholeBodyModel/Kinematics/Forward Kinematics  frameName=Frames.LEFT_FOOT
      settings: SourceProductName=Whole Body Toolbox
  l_sole1 : WBToolboxLibrary/wholeBodyModel/Kinematics/Forward Kinematics  frameName=Frames.LEFT_LEG
      settings: SourceProductName=Whole Body Toolbox
  r_sole : WBToolboxLibrary/wholeBodyModel/Kinematics/Forward Kinematics  frameName=Frames.RIGHT_FOOT
      settings: SourceProductName=Whole Body Toolbox
  r_sole1 : WBToolboxLibrary/wholeBodyModel/Kinematics/Forward Kinematics  frameName=Frames.RIGHT_LEG
      settings: SourceProductName=Whole Body Toolbox
  w_H_lContact : Outport
  w_H_rContact : Outport  Port=2
  JL : Outport  Port=3
  JR : Outport  Port=4
  dJLnu : Outport  Port=5
  dJRnu : Outport  Port=6
  wires:
  r_sole1/1 -> Switch/1
  r_sole/1 -> Switch/3
  l_sole1/1 -> Switch1/1
  l_sole/1 -> Switch1/3
  Switch1/1 -> w_H_lContact/1
  Switch/1 -> w_H_rContact/1
  w_H_b/1 -> Jacobian l_sole1/1, "DotJ Nu l_sole "/1, DotJ Nu l_sole 1/1, "    "/1, " "/1, Jacobian l_sole/1, Jacobian r_sole/1, Jacobian r_sole1/1, r_sole1/1, l_sole/1, l_sole1/1, r_sole/1
  Jacobian r_sole1/1 -> Switch2/1
  legsInContact/1 -> Switch1/2, Switch/2, Switch5/2, Switch4/2, Switch3/2, Switch2/2
  Jacobian r_sole/1 -> Switch2/3
  Jacobian l_sole1/1 -> Switch3/1
  Jacobian l_sole/1 -> Switch3/3
  Switch2/1 -> JR/1
  Switch3/1 -> JL/1
  qj/1 -> l_sole/2, "DotJ Nu l_sole "/2, DotJ Nu l_sole 1/2, "    "/2, " "/2, Jacobian l_sole/2, Jacobian l_sole1/2, Jacobian r_sole/2, Jacobian r_sole1/2, r_sole1/2, r_sole/2, l_sole1/2
  nu_b/1 -> "DotJ Nu l_sole "/3, DotJ Nu l_sole 1/3, "    "/3, " "/3
  dqj/1 -> "DotJ Nu l_sole "/4, DotJ Nu l_sole 1/4, " "/4, "    "/4
  " "/1 -> Switch4/1
  "    "/1 -> Switch4/3
  DotJ Nu l_sole 1/1 -> Switch5/1
  Switch4/1 -> dJRnu/1
  Switch5/1 -> dJLnu/1
  "DotJ Nu l_sole "/1 -> Switch5/3

== system torqueBalancingStandup/Robot system/Dynamics and Kinematics/Kinematics/xCom ==
  w_H_b : Inport
  qj : Inport  Port=2
  CoM : WBToolboxLibrary/wholeBodyModel/Kinematics/Forward Kinematics  frameName=Frames.COM
      settings: SourceProductName=Whole Body Toolbox
  "CoM6D ->  CoMXYZ2" : Selector  NumberOfDimensions=2  InputPortWidth=7  IndexOptions=Index vector (dialog),Index vector (dialog)  Indices=[1 2 3],[4]  OutputSizes=1,1
  xCoM : Outport
  wires:
  qj/1 -> CoM/2
  "CoM6D ->  CoMXYZ2"/1 -> xCoM/1
  CoM/1 -> "CoM6D ->  CoMXYZ2"/1
  w_H_b/1 -> CoM/1

== system torqueBalancingStandup/Robot system/Robot State and References/Internal Coordinator/Base to fixed_link ==
  qj : Inport
  inertial : Inport  Port=2
  Constant1 : Constant  Value=Config.LEFT_FOOT_IN_CONTACT_AT_0
  Constant7 : Constant  Value=eye(4)
  "LFoot to base link transform " : Subsystem
  LFoot to world transform (fixed base) : WBToolboxLibrary/wholeBodyModel/Kinematics/Forward Kinematics  frameName=Frames.LEFT_FOOT
      settings: SourceProductName=Whole Body Toolbox
  RFoot to world transform (fixed base) : WBToolboxLibrary/wholeBodyModel/Kinematics/Forward Kinematics  frameName=Frames.RIGHT_FOOT
      settings: SourceProductName=Whole Body Toolbox
  Switch : Switch  Criteria=u2 > Threshold
  fixed_LFoot_H_b : Outport
  wires:
  "LFoot to base link transform "/1(link_H_b) -> fixed_LFoot_H_b/1
  inertial/1 -> "LFoot to base link transform "/2(inertial)
  qj/1 -> "LFoot to base link transform "/1(qj), RFoot to world transform (fixed base)/2, LFoot to world transform (fixed base)/2
  Constant7/1 -> LFoot to world transform (fixed base)/1, RFoot to world transform (fixed base)/1, "LFoot to base link transform "/4(w_H_base_fixed)
  Switch/1 -> "LFoot to base link transform "/3(w_H_link)
  LFoot to world transform (fixed base)/1 -> Switch/1
  RFoot to world transform (fixed base)/1 -> Switch/3
  Constant1/1 -> Switch/2

== system torqueBalancingStandup/Robot system/Robot State and References/Internal Coordinator/Compute State Velocity ==
  qj : Inport
  w_H_b : Inport  Port=2
  "feetInContact " : Inport  Port=3
  Compute Base Velocity : MATLAB Function  TreatAsAtomicUnit=on
  Feet Jacobians : Subsystem
  Get Measurement : WBToolboxLibrary/wholeBodyStates/Get Measurement  measuredType=Joints Velocity
      settings: SourceProductName=Whole Body Toolbox
  Mux : Mux  Inputs=2
  nu : Outport
  wires:
  Get Measurement/1 -> Mux/2, Compute Base Velocity/4(qjDot)
  Mux/1 -> nu/1
  "feetInContact "/1 -> Compute Base Velocity/3(feetInContact)
  Compute Base Velocity/1(nu_b) -> Mux/1
  qj/1 -> Feet Jacobians/1(qj)
  w_H_b/1 -> Feet Jacobians/2(w_H_b)
  Feet Jacobians/1(J_LFoot) -> Compute Base Velocity/1(J_LeftFoot)
  Feet Jacobians/2(J_RFoot) -> Compute Base Velocity/2(J_RightFoot)

== system torqueBalancingStandup/Robot system/Robot State and References/Internal Coordinator/xCom ==
  w_H_b : Inport
  qj : Inport  Port=2
  CoM : WBToolboxLibrary/wholeBodyModel/Kinematics/Forward Kinematics  frameName=Frames.COM
      settings: SourceProductName=Whole Body Toolbox
  "CoM6D ->  CoMXYZ2" : Selector  NumberOfDimensions=2  InputPortWidth=7  IndexOptions=Index vector (dialog),Index vector (dialog)  Indices=[1 2 3],[4]  OutputSizes=1,1
  xCoM : Outport
  wires:
  qj/1 -> CoM/2
  "CoM6D ->  CoMXYZ2"/1 -> xCoM/1
  CoM/1 -> "CoM6D ->  CoMXYZ2"/1
  w_H_b/1 -> CoM/1

== system torqueBalancingStandup/Robot system/Robot State and References/Select State and References/Visualize Gain Tuning   ==
  smoothingTimeComAndJoints : Inport
  LEFT_RIGHT_FOOT_IN_CONTACT : Inport  Port=2
  impedances : Inport  Port=3
  state : Inport  Port=4
  nu : Inport  Port=5
  Enable : EnablePort
  Demux : Demux  Outputs=2
  DoFs converter : WBToolboxLibrary/Utilities/DoFs converter  Commented=on  yarp2WBIOption=From YARP to WBI
      settings: SourceProductName=Whole Body Toolbox
  DoFs converter1 : WBToolboxLibrary/Utilities/DoFs converter  Commented=on  yarp2WBIOption=From YARP to WBI
      settings: SourceProductName=Whole Body Toolbox
  Gain : Gain  Gain=180/pi
  Gain1 : Gain  Gain=180/pi
  Impedances(t) : Scope  Commented=on  NumInputPorts=6
  Left right foot in contact : Scope
  Selector1 : Selector  InputPortWidth=6+ROBOT_DOF  IndexOptions=Index vector (dialog)  Indices=[7:6+ROBOT_DOF]  OutputSizes=1
  Selector2 : Selector  InputPortWidth=6+ROBOT_DOF  IndexOptions=Index vector (dialog)  Indices=[1:6]  OutputSizes=1
  jointsSmoothingTime : Scope  NumInputPorts=2
  linear and angular  base velocity : Scope  NumInputPorts=3
  "qjDot(t) " : Scope  Commented=on  NumInputPorts=6
  wires:
  state/1 -> "qjDot(t) "/6, linear and angular  base velocity/3, Impedances(t)/6, jointsSmoothingTime/2  "state"
  LEFT_RIGHT_FOOT_IN_CONTACT/1 -> Left right foot in contact/1  "Left right foot in contact"
  impedances/1 -> DoFs converter/1
  smoothingTimeComAndJoints/1 -> jointsSmoothingTime/1  "smoothingTimeComAndJoints"
  DoFs converter/4 -> Impedances(t)/4  "left_leg"
  DoFs converter/5 -> Impedances(t)/5  "right_leg"
  DoFs converter/3 -> Impedances(t)/3  "right_arm"
  DoFs converter/1 -> Impedances(t)/1  "torso"
  DoFs converter/2 -> Impedances(t)/2  "left_arm"
  Selector1/1 -> Gain/1
  DoFs converter1/4 -> "qjDot(t) "/4  "left_leg"
  DoFs converter1/3 -> "qjDot(t) "/3  "right_arm"
  DoFs converter1/1 -> "qjDot(t) "/1  "torso"
  DoFs converter1/2 -> "qjDot(t) "/2  "left_arm"
  nu/1 -> Selector2/1, Selector1/1
  Selector2/1 -> Demux/1
  Demux/1 -> linear and angular  base velocity/1  "vb"
  Demux/2 -> Gain1/1  "wb"
  Gain/1 -> DoFs converter1/1
  Gain1/1 -> linear and angular  base velocity/2
  DoFs converter1/5 -> "qjDot(t) "/5  "right_leg"

== system torqueBalancingStandup/Robot system/Robot State and References/State Machine Standup/Compute State Velocity ==
  qj : Inport
  w_H_b : Inport  Port=2
  "feetInContact " : Inport  Port=3
  "state " : Inport  Port=4
  Compute Base Velocity : MATLAB Function  TreatAsAtomicUnit=on
  Fixed Links Jacobians : Subsystem
  Get Measurement : WBToolboxLibrary/wholeBodyStates/Get Measurement  measuredType=Joints Velocity
      settings: SourceProductName=Whole Body Toolbox
  Mux : Mux  Inputs=2
  nu : Outport
  wires:
  Get Measurement/1 -> Mux/2, Compute Base Velocity/4(qjDot)
  Mux/1 -> nu/1
  "feetInContact "/1 -> Compute Base Velocity/3(feetInContact)
  Compute Base Velocity/1(nu_b) -> Mux/1
  Fixed Links Jacobians/1(J_LeftFixed) -> Compute Base Velocity/1(J_LeftFixedLink)
  Fixed Links Jacobians/2(J_RightFixed) -> Compute Base Velocity/2(J_RightFixedLink)
  "state "/1 -> Fixed Links Jacobians/1("state ")
  qj/1 -> Fixed Links Jacobians/2(qj)
  w_H_b/1 -> Fixed Links Jacobians/3(w_H_b)

== system torqueBalancingStandup/Robot system/Robot State and References/State Machine Standup/Compute base to fixed link transform ==
  qj : Inport
  inertial : Inport  Port=2
  Constant7 : Constant  Value=eye(4)
  "LFoot to base link transform " : Subsystem
  LFoot to world transform (fixed base) : WBToolboxLibrary/wholeBodyModel/Kinematics/Forward Kinematics  frameName=Frames.LEFT_FOOT
      settings: SourceProductName=Whole Body Toolbox
  LLeg to base link transform : Subsystem
  LLeg to world transform (fixed base) : WBToolboxLibrary/wholeBodyModel/Kinematics/Forward Kinematics  frameName=Frames.LEFT_LEG
      settings: SourceProductName=Whole Body Toolbox
  fixed_LFoot_H_b : Outport
  fixed_LLeg_H_b : Outport  Port=2
  wires:
  Constant7/1 -> LLeg to base link transform/4(w_H_base_fixed), "LFoot to base link transform "/4(w_H_base_fixed), LLeg to world transform (fixed base)/1, LFoot to world transform (fixed base)/1
  LLeg to base link transform/1(link_H_b) -> fixed_LLeg_H_b/1
  "LFoot to base link transform "/1(link_H_b) -> fixed_LFoot_H_b/1
  LFoot to world transform (fixed base)/1 -> "LFoot to base link transform "/3(w_H_link)
  LLeg to world transform (fixed base)/1 -> LLeg to base link transform/3(w_H_link)
  qj/1 -> "LFoot to base link transform "/1(qj), LLeg to base link transform/1(qj), LLeg to world transform (fixed base)/2, LFoot to world transform (fixed base)/2
  inertial/1 -> "LFoot to base link transform "/2(inertial), LLeg to base link transform/2(inertial)

== system torqueBalancingStandup/Robot system/Robot State and References/State Machine Standup/Visualise extrnal wrenches ==
  wL_arm : Inport
  wR_arm : Inport  Port=2
  wL_WBDT : Inport  Port=3
  wR_WBDT : Inport  Port=4
  state : Inport  Port=5
  Enable : EnablePort
  Compute current threshold : MATLAB Function  TreatAsAtomicUnit=on
  Sum : Sum  Inputs=++|
  Sum1 : Sum  Inputs=++|
  left arm ext wrench : Scope  NumInputPorts=3
  left foot ext wrench : Scope  NumInputPorts=3
  right arm ext wrench : Scope  NumInputPorts=3
  right foot ext wrench : Scope  NumInputPorts=3
  sum feet ext wrench : Scope  NumInputPorts=3
  wires:
  wR_WBDT/1 -> Sum/2, right foot ext wrench/1  "wR_WBDT"
  wL_WBDT/1 -> Sum/1, left foot ext wrench/1  "wL_WBDT"
  wR_arm/1 -> right arm ext wrench/1
  wL_arm/1 -> left arm ext wrench/1
  state/1 -> Compute current threshold/1(state), sum feet ext wrench/3, right foot ext wrench/3, left foot ext wrench/3, right arm ext wrench/3, left arm ext wrench/3
  Sum/1 -> sum feet ext wrench/1
  Sum1/1 -> sum feet ext wrench/2
  Compute current threshold/3(thresholdContactLeftFoot) -> left foot ext wrench/2, Sum1/1
  Compute current threshold/4(thresholdContactRightFoot) -> right foot ext wrench/2, Sum1/2
  Compute current threshold/1(thresholdContactLeftHand) -> left arm ext wrench/2
  Compute current threshold/2(thresholdContactRightHand) -> right arm ext wrench/2

== system torqueBalancingStandup/Robot system/Robot State and References/State Machine Standup/xCom ==
  w_H_b : Inport
  qj : Inport  Port=2
  CoM : WBToolboxLibrary/wholeBodyModel/Kinematics/Forward Kinematics  frameName=Frames.COM
      settings: SourceProductName=Whole Body Toolbox
  "CoM6D ->  CoMXYZ2" : Selector  NumberOfDimensions=2  InputPortWidth=7  IndexOptions=Index vector (dialog),Index vector (dialog)  Indices=[1 2 3],[4]  OutputSizes=1,1
  xCoM : Outport
  wires:
  qj/1 -> CoM/2
  "CoM6D ->  CoMXYZ2"/1 -> xCoM/1
  CoM/1 -> "CoM6D ->  CoMXYZ2"/1
  w_H_b/1 -> CoM/1

== system torqueBalancingStandup/Robot system/controller_QP/Compute angular momentum integral/Compute base to fixed link transform ==
  qj : Inport
  inertial : Inport  Port=2
  Constant7 : Constant  Value=eye(4)
  "LFoot to base link transform " : Subsystem
  LFoot to world transform (fixed base) : WBToolboxLibrary/wholeBodyModel/Kinematics/Forward Kinematics  frameName=Frames.LEFT_FOOT
      settings: SourceProductName=Whole Body Toolbox
  LLeg to base link transform : Subsystem
  LLeg to world transform (fixed base) : WBToolboxLibrary/wholeBodyModel/Kinematics/Forward Kinematics  frameName=Frames.LEFT_LEG
      settings: SourceProductName=Whole Body Toolbox
  fixed_LLeg_H_b : Outport
  fixed_LFoot_H_b : Outport  Port=2
  wires:
  Constant7/1 -> LLeg to base link transform/4(w_H_base_fixed), "LFoot to base link transform "/4(w_H_base_fixed), LLeg to world transform (fixed base)/1, LFoot to world transform (fixed base)/1
  LLeg to base link transform/1(link_H_b) -> fixed_LLeg_H_b/1
  "LFoot to base link transform "/1(link_H_b) -> fixed_LFoot_H_b/1
  LFoot to world transform (fixed base)/1 -> "LFoot to base link transform "/3(w_H_link)
  LLeg to world transform (fixed base)/1 -> LLeg to base link transform/3(w_H_link)
  qj/1 -> "LFoot to base link transform "/1(qj), LLeg to base link transform/1(qj), LLeg to world transform (fixed base)/2, LFoot to world transform (fixed base)/2
  inertial/1 -> "LFoot to base link transform "/2(inertial), LLeg to base link transform/2(inertial)
